simulink library "Mechanical_Library"  (R2014a)
settings: Solver=ode15s  StartTime=0.0  StopTime=10.0  RelTol=1e-3
libraries: fl_lib x2
settings Model: Creator=ssekkai  LastModifiedBy=ssekkai

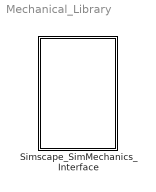
== system Mechanical_Library ==
  Simscape_SimMechanics_Interface : Subsystem

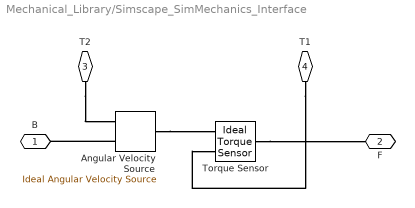
== system Mechanical_Library/Simscape_SimMechanics_Interface ==
  Angular Velocity Source : fl_lib/Mechanical/Mechanical Sources/Ideal Angular Velocity Source
  Torque Sensor : fl_lib/Mechanical/Mechanical Sensors/Ideal Torque Sensor
  B : PMIOPort  Port=1  Side=Left
  F : PMIOPort  Port=2  Side=Left
  T2 : PMIOPort  Port=3  Side=Left
  T1 : PMIOPort  Port=4  Side=Right
  connections:
  T1/RConn1 -- Torque Sensor/RConn2
  T2/RConn1 -- Angular Velocity Source/RConn1
  Torque Sensor/LConn1 -- F/RConn1
  Angular Velocity Source/RConn2 -- B/RConn1
  Angular Velocity Source/LConn1 -- Torque Sensor/RConn1
